simulink model "LQR_crane"  (R2024b)
settings: Solver=ode15s  StartTime=0.0  StopTime=100  MaxStep=1e-3  RelTol=1e-3
values from neighbouring files (symbols this model uses):
  A = [MatriX11, MatriX12, MatriX13, MatriX14, MatriX15, MatriX16,  MatriX17, MatriX18, MatriX19, MatriX110, MatriX111, MatriX112 ... (first row only)    [jacobian_crane.m]    (also in matrices_jacobian.mat = [0 0 0 0 0 0 1 0 0 0 0 0 ... (144 elements, 12x12)]; matrices_jacobian_better.mat = [0 0 0 0 0 0 1 0 0 0 0 0 ... (144 elements, 12x12)])
  B = [0.00067268568898 0 0 0 -0.00401196580412 0 0 0 0 0 0 0 ... (48 elements, 12x4)]    [Bjacobian.mat]    (also in jacobian_crane.m = [B11, B12, B13, B14; matrices_jacobian.mat; matrices_jacobian_better.mat)
  C = eye(12)    [Extended_kalman_filter.m]    (also in crane_control_21_05.m; crane_controlling.m; crane_inner_loop.m = [ 2*d6*dd6*m - dth2*l_B^2*m*sin(2*th2) - dth3*l_J^2*m*sin(2*)
  C_dague = pinv(C)    [crane_control_21_05.m]
  D = zeros(12, 4)    [Extended_kalman_filter.m]    (also in crane_control_21_05.m; crane_controlling.m)
  K = lqr(Ai, Bi, Q, R)    [Extended_kalman_filter.m]    (also in crane_control_21_05.m = lqr(A, B, Q, R); crane_controlling.m = lqr(A, B, Q, R))
  Matrix_pos = diag([zeros(1, floor(12/2)), ones(1, ceil(12/2))])    [crane_control_21_05.m]
  Matrix_speed = [eye(6, 12); zeros(6, 12)]    [crane_control_21_05.m]
  N = K*C_dague - B_dague * A * C_dague    [crane_control_21_05.m]
  x0 = x_eq    [crane_PFL_22_05.m]    (also in crane_control_21_05.m)
  x_d = [0 ... (first row only)    [crane_PFL_22_05.m]    (also in crane_control_21_05.m; crane_controlling.m)
  x_eq = xtraj(1:end, i)    [Extended_kalman_filter.m]    (also in crane_PFL_22_05.m = [zeros(6,1); pi/6; pi/3; -pi/6; 0.5; 0; 0]; crane_control_21_05.m = [zeros(6,1); pi/6; pi/3; -pi/6; 0.5; 0; 0]; crane_controlling.m = [zeros(6,1); pi/6; pi/3; -pi/6; 0.5; 0; 0]; jacobian_crane.m = [zeros(6,1); pi/6; pi/3; -pi/6; 0.5; 0; 0])
settings Model: Creator=david  LastModifiedBy=joelm
settings RTWCC: GPUComputeCapability=3.5

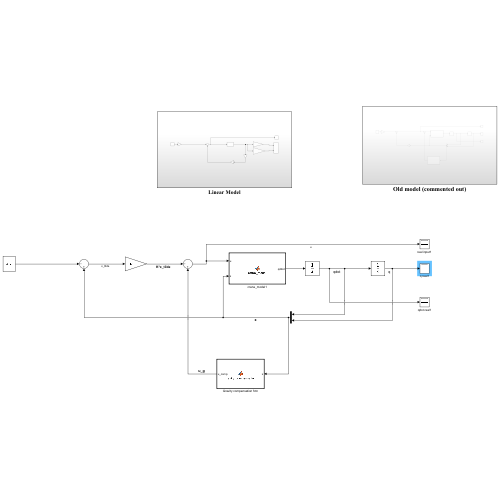
[thumbnail: Simulink's stored preview of the top-level diagram]
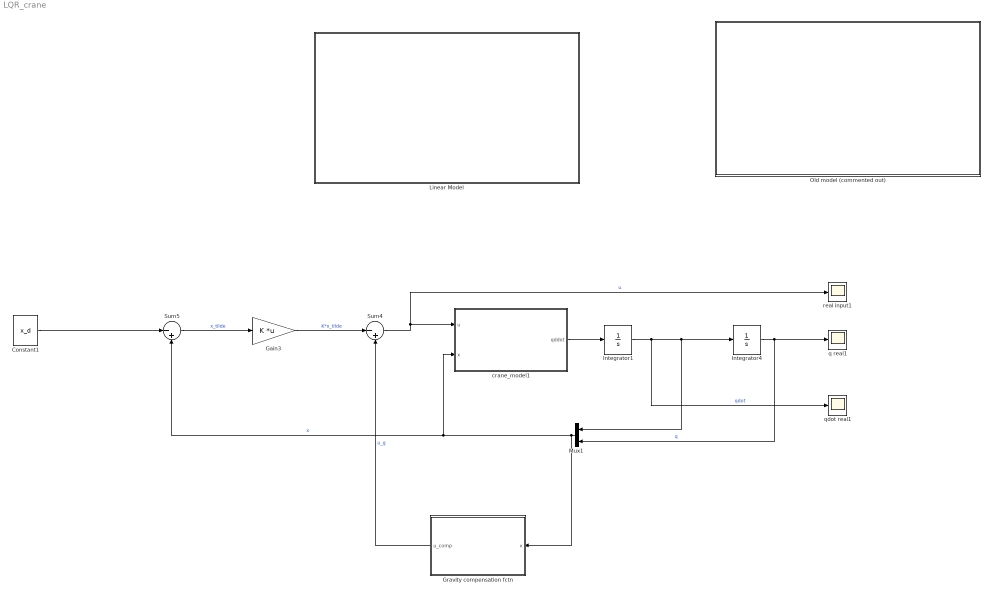
== system LQR_crane ==
  Constant1 : Constant  Value=x_d
  Gain3 : Gain  Gain=K  Multiplication=Matrix(K*u)
  Gravity compensation fctn : MATLAB Function  TreatAsAtomicUnit=on
  Integrator1 : Integrator  InitialCondition=zeros(6,1)
  Integrator4 : Integrator  InitialCondition=x_eq(7:12)
  Linear Model : Subsystem
  Mux1 : Mux  Inputs=2
  Old model (commented out) : Subsystem
  Sum4 : Sum  Inputs=|-+
  Sum5 : Sum  Inputs=|-+
  crane_model1 : MATLAB Function  TreatAsAtomicUnit=on
  q real1 : Scope
  qdot real1 : Scope
  real input1 : Scope
  wires:
  Gravity compensation fctn/1(u_comp) -> Sum4/2  "u_g"
  Sum4/1 -> crane_model1/1(u), real input1/1  "u"
  Integrator4/1 -> Mux1/2, q real1/1  "q"
  Integrator1/1 -> qdot real1/1, Mux1/1, Integrator4/1  "qdot"
  Mux1/1 -> Gravity compensation fctn/1(x), Sum5/2, crane_model1/2(x)  "x"
  Constant1/1 -> Sum5/1
  crane_model1/1(qddot) -> Integrator1/1
  Sum5/1 -> Gain3/1  "x_tilde"
  Gain3/1 -> Sum4/1  "K*x_tilde"

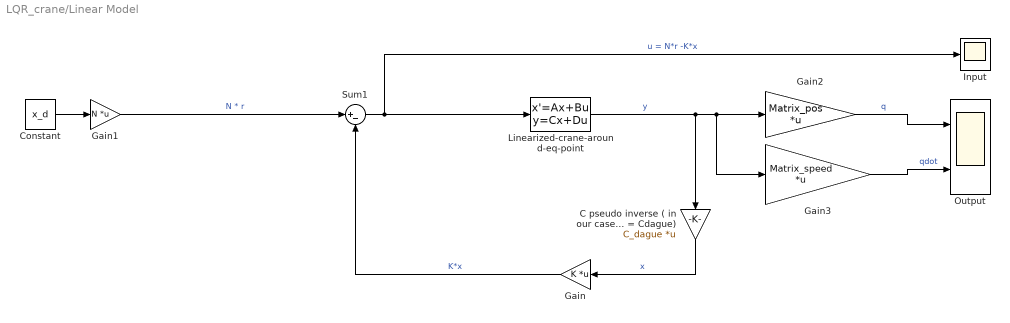
== system LQR_crane/Linear Model ==
  C pseudo inverse ( in our case C is I so = Cdague) : Gain  Gain=C_dague  Multiplication=Matrix(K*u)
  Constant : Constant  Value=x_d
  Gain : Gain  Gain=K  Multiplication=Matrix(K*u)
  Gain1 : Gain  Gain=N  Multiplication=Matrix(K*u)
  Gain2 : Gain  Gain=Matrix_pos  Multiplication=Matrix(K*u)
  Gain3 : Gain  Gain=Matrix_speed  Multiplication=Matrix(K*u)
  Input : Scope
  Linearized-crane-around-eq-point : StateSpace  A=A  B=B  C=C  D=D  InitialCondition=x0
  Output : Scope  NumInputPorts=2
  Sum1 : Sum  Inputs=|+-
  wires:
  Gain/1 -> Sum1/2  "K*x"
  C pseudo inverse ( in our case C is I so = Cdague)/1 -> Gain/1  "x"
  Sum1/1 -> Input/1, Linearized-crane-around-eq-point/1  "u = N*r -K*x"
  Linearized-crane-around-eq-point/1 -> Gain3/1, Gain2/1, C pseudo inverse ( in our case C is I so = Cdague)/1  "y"
  Gain1/1 -> Sum1/1  "N * r"
  Constant/1 -> Gain1/1
  Gain2/1 -> Output/1  "q"
  Gain3/1 -> Output/2  "qdot"

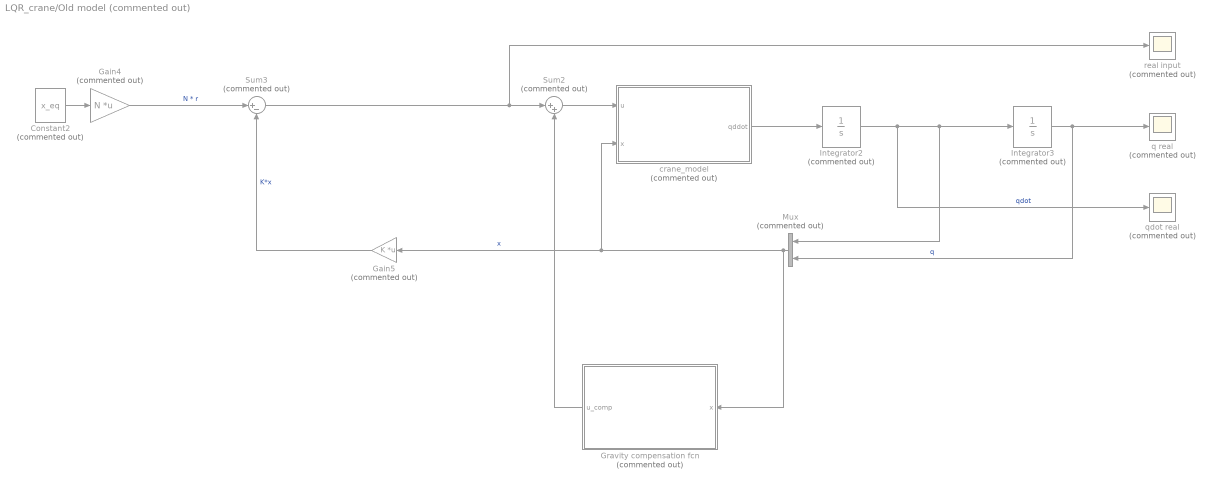
== system LQR_crane/Old model (commented out) ==
  Constant2 : Constant  Commented=on  Value=x_eq
  Gain4 : Gain  Commented=on  Gain=N  Multiplication=Matrix(K*u)
  Gain5 : Gain  Commented=on  Gain=K  Multiplication=Matrix(K*u)
  Gravity compensation fcn : MATLAB Function  Commented=on  TreatAsAtomicUnit=on
  Integrator2 : Integrator  Commented=on  InitialCondition=zeros(6,1)
  Integrator3 : Integrator  Commented=on  InitialCondition=x_eq(7:12)
  Mux : Mux  Commented=on  Inputs=2
  Sum2 : Sum  Commented=on  Inputs=|++
  Sum3 : Sum  Commented=on  Inputs=|+-
  crane_model : MATLAB Function  Commented=on  TreatAsAtomicUnit=on
  q real : Scope  Commented=on
  qdot real : Scope  Commented=on
  real input : Scope  Commented=on
  wires:
  Constant2/1 -> Gain4/1
  Gain5/1 -> Sum3/2  "K*x"
  Sum3/1 -> Sum2/1, real input/1
  Gain4/1 -> Sum3/1  "N * r"
  Mux/1 -> Gravity compensation fcn/1(x), Gain5/1, crane_model/2(x)  "x"
  Integrator3/1 -> Mux/2, q real/1  "q"
  Integrator2/1 -> qdot real/1, Mux/1, Integrator3/1  "qdot"
  Sum2/1 -> crane_model/1(u)
  crane_model/1(qddot) -> Integrator2/1
  Gravity compensation fcn/1(u_comp) -> Sum2/2

== matlab function LQR_crane/Old model (commented out)/Gravity compensation fcn ==
  data: x input; u_comp output
function u_comp = gravity_compensation(x)

I_tot=250;   l_B=2.5;     m_B=300;     I_B=156.25;     l_J=2;     m_J=250;     I_J=85;     g=9.81;       m=90;
  
q = x(7:12);

th1 = q(1);
th2 = q(2);
th3 = q(3);
d6  = q(4);
th4 = q(5);
th5 = q(6);
    
u_comp = [                               0;
(g*l_B*cos(th2)*(2*m + m_B + 2*m_J))/2;
     (g*l_J*cos(th3)*(2*m + m_J))/2;
             -g*m*cos(th4)*cos(th5)];

end

== matlab function LQR_crane/Gravity compensation fctn ==
  data: x input; u_comp output
function u_comp = gravity_compensation(x)

I_tot=250;   l_B=2.5;     m_B=300;     I_B=156.25;     l_J=2;     m_J=250;     I_J=85;     g=9.81;       m=90;
  
q = x(7:12);

th1 = q(1);
th2 = q(2);
th3 = q(3);
d6  = q(4);
th4 = q(5);
th5 = q(6);
    
u_comp = [                               0;
(g*l_B*cos(th2)*(2*m + m_B + 2*m_J))/2;
     (g*l_J*cos(th3)*(2*m + m_J))/2;
             -g*m*cos(th4)*cos(th5)];

end

== matlab function LQR_crane/crane_model1 ==
  data: u input; qddot output; x input
function qddot = crane_model(u, x)



    I_tot=250;   l_B=2.5;     m_B=300;     I_B=156.25;     l_J=2;     m_J=250;     I_J=85;     g=9.81;       m=90;
    
    qdot = x(1:6);
    q = x(7:12); % Function changed for consistency, one state vector with [qdot; q]

    th1 = q(1);
    th2 = q(2);
    th3 = q(3);
    d6  = q(4);
    th4 = q(5);
    th5 = q(6);
    
    
    dth1 = qdot(1);
    dth2 = qdot(2);
    dth3 = qdot(3);
    dd6  =  qdot(4);
    dth4 = qdot(5);
    dth5  =qdot(6);
    
    
    
    M = [ I_tot + d6^2*m + l_B^2*m*cos(th2)^2 + l_J^2*m*cos(th3)^2 + (l_B^2*m_B*cos(th2)^2)/4 + l_B^2*m_J*cos(th2)^2 + (l_J^2*m_J*cos(th3)^2)/4 - d6^2*m*cos(th4)^2*cos(th5)^2 + 2*l_B*l_J*m*cos(th2)*cos(th3) + l_B*l_J*m_J*cos(th2)*cos(th3) + 2*d6*l_B*m*cos(th2)*sin(th5) + 2*d6*l_J*m*cos(th3)*sin(th5),                          d6*l_B*m*cos(th5)*sin(th2)*sin(th4),                          d6*l_J*m*cos(th5)*sin(th3)*sin(th4),            m*cos(th5)*sin(th4)*(l_B*cos(th2) + l_J*cos(th3)), d6*m*cos(th4)*cos(th5)*(l_B*cos(th2) + l_J*cos(th3) + d6*sin(th5)), -d6*m*sin(th4)*(d6 + l_B*cos(th2)*sin(th5) + l_J*cos(th3)*sin(th5));
                                                                                                                                                                                                                                                                     d6*l_B*m*cos(th5)*sin(th2)*sin(th4),                    I_B + l_B^2*m + (l_B^2*m_B)/4 + l_B^2*m_J,                       (l_B*l_J*cos(th2 - th3)*(2*m + m_J))/2, - l_B*m*sin(th2)*sin(th5) - l_B*m*cos(th2)*cos(th4)*cos(th5),                                d6*l_B*m*cos(th2)*cos(th5)*sin(th4),          -d6*l_B*m*(cos(th5)*sin(th2) - cos(th2)*cos(th4)*sin(th5));
                                                                                                                                                                                                                                                                    d6*l_J*m*cos(th5)*sin(th3)*sin(th4),                       (l_B*l_J*cos(th2 - th3)*(2*m + m_J))/2,                                I_J + l_J^2*m + (l_J^2*m_J)/4, - l_J*m*sin(th3)*sin(th5) - l_J*m*cos(th3)*cos(th4)*cos(th5),                                d6*l_J*m*cos(th3)*cos(th5)*sin(th4),          -d6*l_J*m*(cos(th5)*sin(th3) - cos(th3)*cos(th4)*sin(th5));
                                                                                                                                                                                                                                                      m*cos(th5)*sin(th4)*(l_B*cos(th2) + l_J*cos(th3)), - l_B*m*sin(th2)*sin(th5) - l_B*m*cos(th2)*cos(th4)*cos(th5), - l_J*m*sin(th3)*sin(th5) - l_J*m*cos(th3)*cos(th4)*cos(th5),                                                            m,                                                                  0,                                                                   0;
                                                                                                                                                                                                                                     d6*m*cos(th4)*cos(th5)*(l_B*cos(th2) + l_J*cos(th3) + d6*sin(th5)),                          d6*l_B*m*cos(th2)*cos(th5)*sin(th4),                          d6*l_J*m*cos(th3)*cos(th5)*sin(th4),                                                            0,                                           -d6^2*m*(sin(th5)^2 - 1),                                                                   0;
                                                                                                                                                                                                                                    -d6*m*sin(th4)*(d6 + l_B*cos(th2)*sin(th5) + l_J*cos(th3)*sin(th5)),   -d6*l_B*m*(cos(th5)*sin(th2) - cos(th2)*cos(th4)*sin(th5)),   -d6*l_J*m*(cos(th5)*sin(th3) - cos(th3)*cos(th4)*sin(th5)),                                                            0,                                                                  0,                                                              d6^2*m];
                                                                                                                                                                                                                            
    
    % Small regularization
    %%%%%%%%%%%%%%%%%%%%%%%%%%%%%%%%%%%%%%%
    
    C = [ 2*d6*dd6*m - dth2*l_B^2*m*sin(2*th2) - dth3*l_J^2*m*sin(2*th3) - (dth2*l_B^2*m_B*sin(2*th2))/4 - dth2*l_B^2*m_J*sin(2*th2) - (dth3*l_J^2*m_J*sin(2*th3))/4 - 2*d6*dd6*m*cos(th4)^2*cos(th5)^2 + 2*dd6*l_B*m*cos(th2)*sin(th5) + 2*dd6*l_J*m*cos(th3)*sin(th5) + 2*d6*dth5*l_B*m*cos(th2)*cos(th5) + 2*d6*dth5*l_J*m*cos(th3)*cos(th5) - 2*dth2*l_B*l_J*m*cos(th3)*sin(th2) - 2*dth3*l_B*l_J*m*cos(th2)*sin(th3) - dth2*l_B*l_J*m_J*cos(th3)*sin(th2) - dth3*l_B*l_J*m_J*cos(th2)*sin(th3) - 2*d6*dth2*l_B*m*sin(th2)*sin(th5) - 2*d6*dth3*l_J*m*sin(th3)*sin(th5) + 2*d6^2*dth4*m*cos(th4)*cos(th5)^2*sin(th4) + 2*d6^2*dth5*m*cos(th4)^2*cos(th5)*sin(th5),                                                                                                                                                                                                                                                         dd6*l_B*m*cos(th5)*sin(th2)*sin(th4) + d6*dth2*l_B*m*cos(th2)*cos(th5)*sin(th4) + d6*dth4*l_B*m*cos(th4)*cos(th5)*sin(th2) - d6*dth5*l_B*m*sin(th2)*sin(th4)*sin(th5),                                                                                                                                                                                                                                                         dd6*l_J*m*cos(th5)*sin(th3)*sin(th4) + d6*dth3*l_J*m*cos(th3)*cos(th5)*sin(th4) + d6*dth4*l_J*m*cos(th4)*cos(th5)*sin(th3) - d6*dth5*l_J*m*sin(th3)*sin(th4)*sin(th5),       dth4*l_B*m*cos(th2)*cos(th4)*cos(th5) + dth4*l_J*m*cos(th3)*cos(th4)*cos(th5) - dth2*l_B*m*cos(th5)*sin(th2)*sin(th4) - dth5*l_B*m*cos(th2)*sin(th4)*sin(th5) - dth3*l_J*m*cos(th5)*sin(th3)*sin(th4) - dth5*l_J*m*cos(th3)*sin(th4)*sin(th5), 2*d6^2*dth5*m*cos(th4)*cos(th5)^2 - d6^2*dth5*m*cos(th4) + dd6*l_B*m*cos(th2)*cos(th4)*cos(th5) + dd6*l_J*m*cos(th3)*cos(th4)*cos(th5) + 2*d6*dd6*m*cos(th4)*cos(th5)*sin(th5) - d6^2*dth4*m*cos(th5)*sin(th4)*sin(th5) - d6*dth2*l_B*m*cos(th4)*cos(th5)*sin(th2) - d6*dth4*l_B*m*cos(th2)*cos(th5)*sin(th4) - d6*dth5*l_B*m*cos(th2)*cos(th4)*sin(th5) - d6*dth3*l_J*m*cos(th4)*cos(th5)*sin(th3) - d6*dth4*l_J*m*cos(th3)*cos(th5)*sin(th4) - d6*dth5*l_J*m*cos(th3)*cos(th4)*sin(th5), d6*dth2*l_B*m*sin(th2)*sin(th4)*sin(th5) - d6^2*dth4*m*cos(th4) - dd6*l_B*m*cos(th2)*sin(th4)*sin(th5) - dd6*l_J*m*cos(th3)*sin(th4)*sin(th5) - d6*dth4*l_B*m*cos(th2)*cos(th4)*sin(th5) - d6*dth5*l_B*m*cos(th2)*cos(th5)*sin(th4) - d6*dth4*l_J*m*cos(th3)*cos(th4)*sin(th5) - d6*dth5*l_J*m*cos(th3)*cos(th5)*sin(th4) - 2*d6*dd6*m*sin(th4) + d6*dth3*l_J*m*sin(th3)*sin(th4)*sin(th5);
                                                                                                                                                                                                                                                     (dth1*l_B^2*m*sin(2*th2))/2 + (dth1*l_B^2*m_B*sin(2*th2))/8 + (dth1*l_B^2*m_J*sin(2*th2))/2 + (3*dd6*l_B*m*cos(th5)*sin(th2)*sin(th4))/2 + dth1*l_B*l_J*m*cos(th3)*sin(th2) + (dth1*l_B*l_J*m_J*cos(th3)*sin(th2))/2 + d6*dth1*l_B*m*sin(th2)*sin(th5) + (d6*dth2*l_B*m*cos(th2)*cos(th5)*sin(th4))/2 + (3*d6*dth4*l_B*m*cos(th4)*cos(th5)*sin(th2))/2 - (3*d6*dth5*l_B*m*sin(th2)*sin(th4)*sin(th5))/2, (dd6*l_B*m*cos(th2)*sin(th5))/2 - (dd6*l_B*m*cos(th4)*cos(th5)*sin(th2))/2 + (d6*dth5*l_B*m*cos(th2)*cos(th5))/2 - (dth3*l_B*l_J*m*cos(th2)*sin(th3))/2 + (dth3*l_B*l_J*m*cos(th3)*sin(th2))/2 - (dth3*l_B*l_J*m_J*cos(th2)*sin(th3))/4 + (dth3*l_B*l_J*m_J*cos(th3)*sin(th2))/4 - (d6*dth1*l_B*m*cos(th2)*cos(th5)*sin(th4))/2 + (d6*dth4*l_B*m*cos(th5)*sin(th2)*sin(th4))/2 + (d6*dth5*l_B*m*cos(th4)*sin(th2)*sin(th5))/2,                                                                                                                                                                                                                                                                                                                                                                       -(l_B*l_J*sin(th2 - th3)*(dth2 - 2*dth3)*(2*m + m_J))/4,             (dth2*l_B*m*cos(th4)*cos(th5)*sin(th2))/2 - dth5*l_B*m*cos(th5)*sin(th2) - (dth2*l_B*m*cos(th2)*sin(th5))/2 + dth4*l_B*m*cos(th2)*cos(th5)*sin(th4) + dth5*l_B*m*cos(th2)*cos(th4)*sin(th5) + (dth1*l_B*m*cos(th5)*sin(th2)*sin(th4))/2,                                                                                                                                                                                                                                                                  dd6*l_B*m*cos(th2)*cos(th5)*sin(th4) + d6*dth4*l_B*m*cos(th2)*cos(th4)*cos(th5) + (d6*dth1*l_B*m*cos(th4)*cos(th5)*sin(th2))/2 - (d6*dth2*l_B*m*cos(th5)*sin(th2)*sin(th4))/2 - d6*dth5*l_B*m*cos(th2)*sin(th4)*sin(th5),                                                             dd6*l_B*m*cos(th2)*cos(th4)*sin(th5) - dd6*l_B*m*cos(th5)*sin(th2) - (d6*dth2*l_B*m*cos(th2)*cos(th5))/2 + d6*dth5*l_B*m*sin(th2)*sin(th5) + d6*dth5*l_B*m*cos(th2)*cos(th4)*cos(th5) - (d6*dth2*l_B*m*cos(th4)*sin(th2)*sin(th5))/2 - d6*dth4*l_B*m*cos(th2)*sin(th4)*sin(th5) - (d6*dth1*l_B*m*sin(th2)*sin(th4)*sin(th5))/2;
                                                                                                                                                                                                                                                                                     (dth1*l_J^2*m*sin(2*th3))/2 + (dth1*l_J^2*m_J*sin(2*th3))/8 + (3*dd6*l_J*m*cos(th5)*sin(th3)*sin(th4))/2 + dth1*l_B*l_J*m*cos(th2)*sin(th3) + (dth1*l_B*l_J*m_J*cos(th2)*sin(th3))/2 + d6*dth1*l_J*m*sin(th3)*sin(th5) + (d6*dth3*l_J*m*cos(th3)*cos(th5)*sin(th4))/2 + (3*d6*dth4*l_J*m*cos(th4)*cos(th5)*sin(th3))/2 - (3*d6*dth5*l_J*m*sin(th3)*sin(th4)*sin(th5))/2,                                                                                                                                                                                                                                                                                                                                                                       -(l_B*l_J*sin(th2 - th3)*(2*m + m_J)*(2*dth2 - dth3))/4, (dd6*l_J*m*cos(th3)*sin(th5))/2 - (dd6*l_J*m*cos(th4)*cos(th5)*sin(th3))/2 + (d6*dth5*l_J*m*cos(th3)*cos(th5))/2 + (dth2*l_B*l_J*m*cos(th2)*sin(th3))/2 - (dth2*l_B*l_J*m*cos(th3)*sin(th2))/2 + (dth2*l_B*l_J*m_J*cos(th2)*sin(th3))/4 - (dth2*l_B*l_J*m_J*cos(th3)*sin(th2))/4 - (d6*dth1*l_J*m*cos(th3)*cos(th5)*sin(th4))/2 + (d6*dth4*l_J*m*cos(th5)*sin(th3)*sin(th4))/2 + (d6*dth5*l_J*m*cos(th4)*sin(th3)*sin(th5))/2,             (dth3*l_J*m*cos(th4)*cos(th5)*sin(th3))/2 - dth5*l_J*m*cos(th5)*sin(th3) - (dth3*l_J*m*cos(th3)*sin(th5))/2 + dth4*l_J*m*cos(th3)*cos(th5)*sin(th4) + dth5*l_J*m*cos(th3)*cos(th4)*sin(th5) + (dth1*l_J*m*cos(th5)*sin(th3)*sin(th4))/2,                                                                                                                                                                                                                                                                  dd6*l_J*m*cos(th3)*cos(th5)*sin(th4) + d6*dth4*l_J*m*cos(th3)*cos(th4)*cos(th5) + (d6*dth1*l_J*m*cos(th4)*cos(th5)*sin(th3))/2 - (d6*dth3*l_J*m*cos(th5)*sin(th3)*sin(th4))/2 - d6*dth5*l_J*m*cos(th3)*sin(th4)*sin(th5),                                                             dd6*l_J*m*cos(th3)*cos(th4)*sin(th5) - dd6*l_J*m*cos(th5)*sin(th3) - (d6*dth3*l_J*m*cos(th3)*cos(th5))/2 + d6*dth5*l_J*m*sin(th3)*sin(th5) + d6*dth5*l_J*m*cos(th3)*cos(th4)*cos(th5) - (d6*dth3*l_J*m*cos(th4)*sin(th3)*sin(th5))/2 - d6*dth4*l_J*m*cos(th3)*sin(th4)*sin(th5) - (d6*dth1*l_J*m*sin(th3)*sin(th4)*sin(th5))/2;
                                                                                                                                                                                                           d6*dth5*m*sin(th4) - d6*dth1*m + d6*dth1*m*cos(th4)^2*cos(th5)^2 - dth1*l_B*m*cos(th2)*sin(th5) - dth1*l_J*m*cos(th3)*sin(th5) + (dth4*l_B*m*cos(th2)*cos(th4)*cos(th5))/2 + (dth4*l_J*m*cos(th3)*cos(th4)*cos(th5))/2 - d6*dth4*m*cos(th4)*cos(th5)*sin(th5) - (3*dth2*l_B*m*cos(th5)*sin(th2)*sin(th4))/2 - (dth5*l_B*m*cos(th2)*sin(th4)*sin(th5))/2 - (3*dth3*l_J*m*cos(th5)*sin(th3)*sin(th4))/2 - (dth5*l_J*m*cos(th3)*sin(th4)*sin(th5))/2,                                                                                                                                                                                   dth2*l_B*m*cos(th4)*cos(th5)*sin(th2) - (dth5*l_B*m*cos(th5)*sin(th2))/2 - dth2*l_B*m*cos(th2)*sin(th5) + (dth4*l_B*m*cos(th2)*cos(th5)*sin(th4))/2 + (dth5*l_B*m*cos(th2)*cos(th4)*sin(th5))/2 - (dth1*l_B*m*cos(th5)*sin(th2)*sin(th4))/2,                                                                                                                                                                                   dth3*l_J*m*cos(th4)*cos(th5)*sin(th3) - (dth5*l_J*m*cos(th5)*sin(th3))/2 - dth3*l_J*m*cos(th3)*sin(th5) + (dth4*l_J*m*cos(th3)*cos(th5)*sin(th4))/2 + (dth5*l_J*m*cos(th3)*cos(th4)*sin(th5))/2 - (dth1*l_J*m*cos(th5)*sin(th3)*sin(th4))/2,                                                                                                                                                                                                                                                   0,                                                                                                                                                                                                                                                                                                    -(m*cos(th5)*(2*d6*dth4*cos(th5) + dth1*l_B*cos(th2)*cos(th4) + dth1*l_J*cos(th3)*cos(th4) + 2*d6*dth1*cos(th4)*sin(th5) + dth2*l_B*cos(th2)*sin(th4) + dth3*l_J*cos(th3)*sin(th4)))/2,                                                                                                       d6*dth1*m*sin(th4) - d6*dth5*m + (dth2*l_B*m*cos(th5)*sin(th2))/2 + (dth3*l_J*m*cos(th5)*sin(th3))/2 - (dth2*l_B*m*cos(th2)*cos(th4)*sin(th5))/2 - (dth3*l_J*m*cos(th3)*cos(th4)*sin(th5))/2 + (dth1*l_B*m*cos(th2)*sin(th4)*sin(th5))/2 + (dth1*l_J*m*cos(th3)*sin(th4)*sin(th5))/2;
                                                                            2*d6^2*dth5*m*cos(th4)*cos(th5)^2 - (d6^2*dth5*m*cos(th4))/2 + (dd6*l_B*m*cos(th2)*cos(th4)*cos(th5))/2 + (dd6*l_J*m*cos(th3)*cos(th4)*cos(th5))/2 + 2*d6*dd6*m*cos(th4)*cos(th5)*sin(th5) - (d6^2*dth4*m*cos(th5)*sin(th4)*sin(th5))/2 - d6^2*dth1*m*cos(th4)*cos(th5)^2*sin(th4) - (3*d6*dth2*l_B*m*cos(th4)*cos(th5)*sin(th2))/2 - (d6*dth4*l_B*m*cos(th2)*cos(th5)*sin(th4))/2 - (d6*dth5*l_B*m*cos(th2)*cos(th4)*sin(th5))/2 - (3*d6*dth3*l_J*m*cos(th4)*cos(th5)*sin(th3))/2 - (d6*dth4*l_J*m*cos(th3)*cos(th5)*sin(th4))/2 - (d6*dth5*l_J*m*cos(th3)*cos(th4)*sin(th5))/2,                                                                                                                                                                                              (dd6*l_B*m*cos(th2)*cos(th5)*sin(th4))/2 + (d6*dth4*l_B*m*cos(th2)*cos(th4)*cos(th5))/2 - (d6*dth1*l_B*m*cos(th4)*cos(th5)*sin(th2))/2 - d6*dth2*l_B*m*cos(th5)*sin(th2)*sin(th4) - (d6*dth5*l_B*m*cos(th2)*sin(th4)*sin(th5))/2,                                                                                                                                                                                              (dd6*l_J*m*cos(th3)*cos(th5)*sin(th4))/2 + (d6*dth4*l_J*m*cos(th3)*cos(th4)*cos(th5))/2 - (d6*dth1*l_J*m*cos(th4)*cos(th5)*sin(th3))/2 - d6*dth3*l_J*m*cos(th5)*sin(th3)*sin(th4) - (d6*dth5*l_J*m*cos(th3)*sin(th4)*sin(th5))/2,                                                                                                                 -(m*cos(th5)*(dth1*l_B*cos(th2)*cos(th4) + dth1*l_J*cos(th3)*cos(th4) + dth2*l_B*cos(th2)*sin(th4) + dth3*l_J*cos(th3)*sin(th4)))/2,                                                                                                                                                                                                                                                                                   (d6*m*cos(th5)*(4*dd6*cos(th5) - 4*d6*dth5*sin(th5) - dth2*l_B*cos(th2)*cos(th4) - dth3*l_J*cos(th3)*cos(th4) + dth1*l_B*cos(th2)*sin(th4) + dth1*l_J*cos(th3)*sin(th4) + d6*dth1*sin(th4)*sin(th5)))/2,                                                                                                                                                                                                        (d6*m*(d6*dth1*cos(th4) + dth1*l_B*cos(th2)*cos(th4)*sin(th5) + dth1*l_J*cos(th3)*cos(th4)*sin(th5) + dth2*l_B*cos(th2)*sin(th4)*sin(th5) + dth3*l_J*cos(th3)*sin(th4)*sin(th5)))/2;
                                                                         (3*d6*dth2*l_B*m*sin(th2)*sin(th4)*sin(th5))/2 - (d6^2*dth4*m*cos(th4))/2 - d6^2*dth4*m*cos(th4)*cos(th5)^2 - (dd6*l_B*m*cos(th2)*sin(th4)*sin(th5))/2 - (dd6*l_J*m*cos(th3)*sin(th4)*sin(th5))/2 - d6*dth1*l_B*m*cos(th2)*cos(th5) - d6*dth1*l_J*m*cos(th3)*cos(th5) - d6^2*dth1*m*cos(th4)^2*cos(th5)*sin(th5) - (d6*dth4*l_B*m*cos(th2)*cos(th4)*sin(th5))/2 - (d6*dth5*l_B*m*cos(th2)*cos(th5)*sin(th4))/2 - (d6*dth4*l_J*m*cos(th3)*cos(th4)*sin(th5))/2 - (d6*dth5*l_J*m*cos(th3)*cos(th5)*sin(th4))/2 - 2*d6*dd6*m*sin(th4) + (3*d6*dth3*l_J*m*sin(th3)*sin(th4)*sin(th5))/2,                                                                                    (dd6*l_B*m*cos(th2)*cos(th4)*sin(th5))/2 - (dd6*l_B*m*cos(th5)*sin(th2))/2 - d6*dth2*l_B*m*cos(th2)*cos(th5) + (d6*dth5*l_B*m*sin(th2)*sin(th5))/2 + (d6*dth5*l_B*m*cos(th2)*cos(th4)*cos(th5))/2 - d6*dth2*l_B*m*cos(th4)*sin(th2)*sin(th5) - (d6*dth4*l_B*m*cos(th2)*sin(th4)*sin(th5))/2 + (d6*dth1*l_B*m*sin(th2)*sin(th4)*sin(th5))/2,                                                                                    (dd6*l_J*m*cos(th3)*cos(th4)*sin(th5))/2 - (dd6*l_J*m*cos(th5)*sin(th3))/2 - d6*dth3*l_J*m*cos(th3)*cos(th5) + (d6*dth5*l_J*m*sin(th3)*sin(th5))/2 + (d6*dth5*l_J*m*cos(th3)*cos(th4)*cos(th5))/2 - d6*dth3*l_J*m*cos(th4)*sin(th3)*sin(th5) - (d6*dth4*l_J*m*cos(th3)*sin(th4)*sin(th5))/2 + (d6*dth1*l_J*m*sin(th3)*sin(th4)*sin(th5))/2, (dth2*l_B*m*cos(th5)*sin(th2))/2 + (dth3*l_J*m*cos(th5)*sin(th3))/2 - (dth2*l_B*m*cos(th2)*cos(th4)*sin(th5))/2 - (dth3*l_J*m*cos(th3)*cos(th4)*sin(th5))/2 + (dth1*l_B*m*cos(th2)*sin(th4)*sin(th5))/2 + (dth1*l_J*m*cos(th3)*sin(th4)*sin(th5))/2,                                                                                                                                                                                                    (d6^2*dth1*m*cos(th4))/2 - d6^2*dth1*m*cos(th4)*cos(th5)^2 + d6^2*dth4*m*cos(th5)*sin(th5) + (d6*dth1*l_B*m*cos(th2)*cos(th4)*sin(th5))/2 + (d6*dth1*l_J*m*cos(th3)*cos(th4)*sin(th5))/2 + (d6*dth2*l_B*m*cos(th2)*sin(th4)*sin(th5))/2 + (d6*dth3*l_J*m*cos(th3)*sin(th4)*sin(th5))/2,                                                                                                                                                        -(d6*m*(dth2*l_B*sin(th2)*sin(th5) - 4*dd6 + dth3*l_J*sin(th3)*sin(th5) + dth2*l_B*cos(th2)*cos(th4)*cos(th5) + dth3*l_J*cos(th3)*cos(th4)*cos(th5) - dth1*l_B*cos(th2)*cos(th5)*sin(th4) - dth1*l_J*cos(th3)*cos(th5)*sin(th4)))/2];
    
    
    %%%%%%%%%%%%%%%%%%%%%%%%%%%%%%%%%%%%%%%%%%%%%
    
    G = [                                0;
    (g*l_B*cos(th2)*(2*m + m_B + 2*m_J))/2;
         (g*l_J*cos(th3)*(2*m + m_J))/2;
                 -g*m*cos(th4)*cos(th5);
               d6*g*m*cos(th5)*sin(th4);
               d6*g*m*cos(th4)*sin(th5)];

    U = [u(1); u(2); u(3); u(4); 0; 0];     %%%the last two dof are the angles of the swaying cable and are not actuable

    
    % Compute right-hand side
    rhs = -C*qdot - G + U;
    
    % Solve for qddot 
    qddot = M \ rhs;
    
    

end

== matlab function LQR_crane/Old model (commented out)/crane_model ==
  data: u input; qddot output; x input
function qddot = crane_model(u, x)



    I_tot=250;   l_B=2.5;     m_B=300;     I_B=156.25;     l_J=2;     m_J=250;     I_J=85;     g=9.81;       m=90;
    
    qdot = x(1:6);
    q = x(7:12); % Function changed for consistency, one state vector with [qdot; q]

    th1 = q(1);
    th2 = q(2);
    th3 = q(3);
    d6  = q(4);
    th4 = q(5);
    th5 = q(6);
    
    
    dth1 = qdot(1);
    dth2 = qdot(2);
    dth3 = qdot(3);
    dd6  =  qdot(4);
    dth4 = qdot(5);
    dth5  =qdot(6);
    
    
    
    M = [ I_tot + d6^2*m + l_B^2*m*cos(th2)^2 + l_J^2*m*cos(th3)^2 + (l_B^2*m_B*cos(th2)^2)/4 + l_B^2*m_J*cos(th2)^2 + (l_J^2*m_J*cos(th3)^2)/4 - d6^2*m*cos(th4)^2*cos(th5)^2 + 2*l_B*l_J*m*cos(th2)*cos(th3) + l_B*l_J*m_J*cos(th2)*cos(th3) + 2*d6*l_B*m*cos(th2)*sin(th5) + 2*d6*l_J*m*cos(th3)*sin(th5),                          d6*l_B*m*cos(th5)*sin(th2)*sin(th4),                          d6*l_J*m*cos(th5)*sin(th3)*sin(th4),            m*cos(th5)*sin(th4)*(l_B*cos(th2) + l_J*cos(th3)), d6*m*cos(th4)*cos(th5)*(l_B*cos(th2) + l_J*cos(th3) + d6*sin(th5)), -d6*m*sin(th4)*(d6 + l_B*cos(th2)*sin(th5) + l_J*cos(th3)*sin(th5));
                                                                                                                                                                                                                                                                     d6*l_B*m*cos(th5)*sin(th2)*sin(th4),                    I_B + l_B^2*m + (l_B^2*m_B)/4 + l_B^2*m_J,                       (l_B*l_J*cos(th2 - th3)*(2*m + m_J))/2, - l_B*m*sin(th2)*sin(th5) - l_B*m*cos(th2)*cos(th4)*cos(th5),                                d6*l_B*m*cos(th2)*cos(th5)*sin(th4),          -d6*l_B*m*(cos(th5)*sin(th2) - cos(th2)*cos(th4)*sin(th5));
                                                                                                                                                                                                                                                                    d6*l_J*m*cos(th5)*sin(th3)*sin(th4),                       (l_B*l_J*cos(th2 - th3)*(2*m + m_J))/2,                                I_J + l_J^2*m + (l_J^2*m_J)/4, - l_J*m*sin(th3)*sin(th5) - l_J*m*cos(th3)*cos(th4)*cos(th5),                                d6*l_J*m*cos(th3)*cos(th5)*sin(th4),          -d6*l_J*m*(cos(th5)*sin(th3) - cos(th3)*cos(th4)*sin(th5));
                                                                                                                                                                                                                                                      m*cos(th5)*sin(th4)*(l_B*cos(th2) + l_J*cos(th3)), - l_B*m*sin(th2)*sin(th5) - l_B*m*cos(th2)*cos(th4)*cos(th5), - l_J*m*sin(th3)*sin(th5) - l_J*m*cos(th3)*cos(th4)*cos(th5),                                                            m,                                                                  0,                                                                   0;
                                                                                                                                                                                                                                     d6*m*cos(th4)*cos(th5)*(l_B*cos(th2) + l_J*cos(th3) + d6*sin(th5)),                          d6*l_B*m*cos(th2)*cos(th5)*sin(th4),                          d6*l_J*m*cos(th3)*cos(th5)*sin(th4),                                                            0,                                           -d6^2*m*(sin(th5)^2 - 1),                                                                   0;
                                                                                                                                                                                                                                    -d6*m*sin(th4)*(d6 + l_B*cos(th2)*sin(th5) + l_J*cos(th3)*sin(th5)),   -d6*l_B*m*(cos(th5)*sin(th2) - cos(th2)*cos(th4)*sin(th5)),   -d6*l_J*m*(cos(th5)*sin(th3) - cos(th3)*cos(th4)*sin(th5)),                                                            0,                                                                  0,                                                              d6^2*m];
                                                                                                                                                                                                                            
    
    % Small regularization
    %%%%%%%%%%%%%%%%%%%%%%%%%%%%%%%%%%%%%%%
    
    C = [ 2*d6*dd6*m - dth2*l_B^2*m*sin(2*th2) - dth3*l_J^2*m*sin(2*th3) - (dth2*l_B^2*m_B*sin(2*th2))/4 - dth2*l_B^2*m_J*sin(2*th2) - (dth3*l_J^2*m_J*sin(2*th3))/4 - 2*d6*dd6*m*cos(th4)^2*cos(th5)^2 + 2*dd6*l_B*m*cos(th2)*sin(th5) + 2*dd6*l_J*m*cos(th3)*sin(th5) + 2*d6*dth5*l_B*m*cos(th2)*cos(th5) + 2*d6*dth5*l_J*m*cos(th3)*cos(th5) - 2*dth2*l_B*l_J*m*cos(th3)*sin(th2) - 2*dth3*l_B*l_J*m*cos(th2)*sin(th3) - dth2*l_B*l_J*m_J*cos(th3)*sin(th2) - dth3*l_B*l_J*m_J*cos(th2)*sin(th3) - 2*d6*dth2*l_B*m*sin(th2)*sin(th5) - 2*d6*dth3*l_J*m*sin(th3)*sin(th5) + 2*d6^2*dth4*m*cos(th4)*cos(th5)^2*sin(th4) + 2*d6^2*dth5*m*cos(th4)^2*cos(th5)*sin(th5),                                                                                                                                                                                                                                                         dd6*l_B*m*cos(th5)*sin(th2)*sin(th4) + d6*dth2*l_B*m*cos(th2)*cos(th5)*sin(th4) + d6*dth4*l_B*m*cos(th4)*cos(th5)*sin(th2) - d6*dth5*l_B*m*sin(th2)*sin(th4)*sin(th5),                                                                                                                                                                                                                                                         dd6*l_J*m*cos(th5)*sin(th3)*sin(th4) + d6*dth3*l_J*m*cos(th3)*cos(th5)*sin(th4) + d6*dth4*l_J*m*cos(th4)*cos(th5)*sin(th3) - d6*dth5*l_J*m*sin(th3)*sin(th4)*sin(th5),       dth4*l_B*m*cos(th2)*cos(th4)*cos(th5) + dth4*l_J*m*cos(th3)*cos(th4)*cos(th5) - dth2*l_B*m*cos(th5)*sin(th2)*sin(th4) - dth5*l_B*m*cos(th2)*sin(th4)*sin(th5) - dth3*l_J*m*cos(th5)*sin(th3)*sin(th4) - dth5*l_J*m*cos(th3)*sin(th4)*sin(th5), 2*d6^2*dth5*m*cos(th4)*cos(th5)^2 - d6^2*dth5*m*cos(th4) + dd6*l_B*m*cos(th2)*cos(th4)*cos(th5) + dd6*l_J*m*cos(th3)*cos(th4)*cos(th5) + 2*d6*dd6*m*cos(th4)*cos(th5)*sin(th5) - d6^2*dth4*m*cos(th5)*sin(th4)*sin(th5) - d6*dth2*l_B*m*cos(th4)*cos(th5)*sin(th2) - d6*dth4*l_B*m*cos(th2)*cos(th5)*sin(th4) - d6*dth5*l_B*m*cos(th2)*cos(th4)*sin(th5) - d6*dth3*l_J*m*cos(th4)*cos(th5)*sin(th3) - d6*dth4*l_J*m*cos(th3)*cos(th5)*sin(th4) - d6*dth5*l_J*m*cos(th3)*cos(th4)*sin(th5), d6*dth2*l_B*m*sin(th2)*sin(th4)*sin(th5) - d6^2*dth4*m*cos(th4) - dd6*l_B*m*cos(th2)*sin(th4)*sin(th5) - dd6*l_J*m*cos(th3)*sin(th4)*sin(th5) - d6*dth4*l_B*m*cos(th2)*cos(th4)*sin(th5) - d6*dth5*l_B*m*cos(th2)*cos(th5)*sin(th4) - d6*dth4*l_J*m*cos(th3)*cos(th4)*sin(th5) - d6*dth5*l_J*m*cos(th3)*cos(th5)*sin(th4) - 2*d6*dd6*m*sin(th4) + d6*dth3*l_J*m*sin(th3)*sin(th4)*sin(th5);
                                                                                                                                                                                                                                                     (dth1*l_B^2*m*sin(2*th2))/2 + (dth1*l_B^2*m_B*sin(2*th2))/8 + (dth1*l_B^2*m_J*sin(2*th2))/2 + (3*dd6*l_B*m*cos(th5)*sin(th2)*sin(th4))/2 + dth1*l_B*l_J*m*cos(th3)*sin(th2) + (dth1*l_B*l_J*m_J*cos(th3)*sin(th2))/2 + d6*dth1*l_B*m*sin(th2)*sin(th5) + (d6*dth2*l_B*m*cos(th2)*cos(th5)*sin(th4))/2 + (3*d6*dth4*l_B*m*cos(th4)*cos(th5)*sin(th2))/2 - (3*d6*dth5*l_B*m*sin(th2)*sin(th4)*sin(th5))/2, (dd6*l_B*m*cos(th2)*sin(th5))/2 - (dd6*l_B*m*cos(th4)*cos(th5)*sin(th2))/2 + (d6*dth5*l_B*m*cos(th2)*cos(th5))/2 - (dth3*l_B*l_J*m*cos(th2)*sin(th3))/2 + (dth3*l_B*l_J*m*cos(th3)*sin(th2))/2 - (dth3*l_B*l_J*m_J*cos(th2)*sin(th3))/4 + (dth3*l_B*l_J*m_J*cos(th3)*sin(th2))/4 - (d6*dth1*l_B*m*cos(th2)*cos(th5)*sin(th4))/2 + (d6*dth4*l_B*m*cos(th5)*sin(th2)*sin(th4))/2 + (d6*dth5*l_B*m*cos(th4)*sin(th2)*sin(th5))/2,                                                                                                                                                                                                                                                                                                                                                                       -(l_B*l_J*sin(th2 - th3)*(dth2 - 2*dth3)*(2*m + m_J))/4,             (dth2*l_B*m*cos(th4)*cos(th5)*sin(th2))/2 - dth5*l_B*m*cos(th5)*sin(th2) - (dth2*l_B*m*cos(th2)*sin(th5))/2 + dth4*l_B*m*cos(th2)*cos(th5)*sin(th4) + dth5*l_B*m*cos(th2)*cos(th4)*sin(th5) + (dth1*l_B*m*cos(th5)*sin(th2)*sin(th4))/2,                                                                                                                                                                                                                                                                  dd6*l_B*m*cos(th2)*cos(th5)*sin(th4) + d6*dth4*l_B*m*cos(th2)*cos(th4)*cos(th5) + (d6*dth1*l_B*m*cos(th4)*cos(th5)*sin(th2))/2 - (d6*dth2*l_B*m*cos(th5)*sin(th2)*sin(th4))/2 - d6*dth5*l_B*m*cos(th2)*sin(th4)*sin(th5),                                                             dd6*l_B*m*cos(th2)*cos(th4)*sin(th5) - dd6*l_B*m*cos(th5)*sin(th2) - (d6*dth2*l_B*m*cos(th2)*cos(th5))/2 + d6*dth5*l_B*m*sin(th2)*sin(th5) + d6*dth5*l_B*m*cos(th2)*cos(th4)*cos(th5) - (d6*dth2*l_B*m*cos(th4)*sin(th2)*sin(th5))/2 - d6*dth4*l_B*m*cos(th2)*sin(th4)*sin(th5) - (d6*dth1*l_B*m*sin(th2)*sin(th4)*sin(th5))/2;
                                                                                                                                                                                                                                                                                     (dth1*l_J^2*m*sin(2*th3))/2 + (dth1*l_J^2*m_J*sin(2*th3))/8 + (3*dd6*l_J*m*cos(th5)*sin(th3)*sin(th4))/2 + dth1*l_B*l_J*m*cos(th2)*sin(th3) + (dth1*l_B*l_J*m_J*cos(th2)*sin(th3))/2 + d6*dth1*l_J*m*sin(th3)*sin(th5) + (d6*dth3*l_J*m*cos(th3)*cos(th5)*sin(th4))/2 + (3*d6*dth4*l_J*m*cos(th4)*cos(th5)*sin(th3))/2 - (3*d6*dth5*l_J*m*sin(th3)*sin(th4)*sin(th5))/2,                                                                                                                                                                                                                                                                                                                                                                       -(l_B*l_J*sin(th2 - th3)*(2*m + m_J)*(2*dth2 - dth3))/4, (dd6*l_J*m*cos(th3)*sin(th5))/2 - (dd6*l_J*m*cos(th4)*cos(th5)*sin(th3))/2 + (d6*dth5*l_J*m*cos(th3)*cos(th5))/2 + (dth2*l_B*l_J*m*cos(th2)*sin(th3))/2 - (dth2*l_B*l_J*m*cos(th3)*sin(th2))/2 + (dth2*l_B*l_J*m_J*cos(th2)*sin(th3))/4 - (dth2*l_B*l_J*m_J*cos(th3)*sin(th2))/4 - (d6*dth1*l_J*m*cos(th3)*cos(th5)*sin(th4))/2 + (d6*dth4*l_J*m*cos(th5)*sin(th3)*sin(th4))/2 + (d6*dth5*l_J*m*cos(th4)*sin(th3)*sin(th5))/2,             (dth3*l_J*m*cos(th4)*cos(th5)*sin(th3))/2 - dth5*l_J*m*cos(th5)*sin(th3) - (dth3*l_J*m*cos(th3)*sin(th5))/2 + dth4*l_J*m*cos(th3)*cos(th5)*sin(th4) + dth5*l_J*m*cos(th3)*cos(th4)*sin(th5) + (dth1*l_J*m*cos(th5)*sin(th3)*sin(th4))/2,                                                                                                                                                                                                                                                                  dd6*l_J*m*cos(th3)*cos(th5)*sin(th4) + d6*dth4*l_J*m*cos(th3)*cos(th4)*cos(th5) + (d6*dth1*l_J*m*cos(th4)*cos(th5)*sin(th3))/2 - (d6*dth3*l_J*m*cos(th5)*sin(th3)*sin(th4))/2 - d6*dth5*l_J*m*cos(th3)*sin(th4)*sin(th5),                                                             dd6*l_J*m*cos(th3)*cos(th4)*sin(th5) - dd6*l_J*m*cos(th5)*sin(th3) - (d6*dth3*l_J*m*cos(th3)*cos(th5))/2 + d6*dth5*l_J*m*sin(th3)*sin(th5) + d6*dth5*l_J*m*cos(th3)*cos(th4)*cos(th5) - (d6*dth3*l_J*m*cos(th4)*sin(th3)*sin(th5))/2 - d6*dth4*l_J*m*cos(th3)*sin(th4)*sin(th5) - (d6*dth1*l_J*m*sin(th3)*sin(th4)*sin(th5))/2;
                                                                                                                                                                                                           d6*dth5*m*sin(th4) - d6*dth1*m + d6*dth1*m*cos(th4)^2*cos(th5)^2 - dth1*l_B*m*cos(th2)*sin(th5) - dth1*l_J*m*cos(th3)*sin(th5) + (dth4*l_B*m*cos(th2)*cos(th4)*cos(th5))/2 + (dth4*l_J*m*cos(th3)*cos(th4)*cos(th5))/2 - d6*dth4*m*cos(th4)*cos(th5)*sin(th5) - (3*dth2*l_B*m*cos(th5)*sin(th2)*sin(th4))/2 - (dth5*l_B*m*cos(th2)*sin(th4)*sin(th5))/2 - (3*dth3*l_J*m*cos(th5)*sin(th3)*sin(th4))/2 - (dth5*l_J*m*cos(th3)*sin(th4)*sin(th5))/2,                                                                                                                                                                                   dth2*l_B*m*cos(th4)*cos(th5)*sin(th2) - (dth5*l_B*m*cos(th5)*sin(th2))/2 - dth2*l_B*m*cos(th2)*sin(th5) + (dth4*l_B*m*cos(th2)*cos(th5)*sin(th4))/2 + (dth5*l_B*m*cos(th2)*cos(th4)*sin(th5))/2 - (dth1*l_B*m*cos(th5)*sin(th2)*sin(th4))/2,                                                                                                                                                                                   dth3*l_J*m*cos(th4)*cos(th5)*sin(th3) - (dth5*l_J*m*cos(th5)*sin(th3))/2 - dth3*l_J*m*cos(th3)*sin(th5) + (dth4*l_J*m*cos(th3)*cos(th5)*sin(th4))/2 + (dth5*l_J*m*cos(th3)*cos(th4)*sin(th5))/2 - (dth1*l_J*m*cos(th5)*sin(th3)*sin(th4))/2,                                                                                                                                                                                                                                                   0,                                                                                                                                                                                                                                                                                                    -(m*cos(th5)*(2*d6*dth4*cos(th5) + dth1*l_B*cos(th2)*cos(th4) + dth1*l_J*cos(th3)*cos(th4) + 2*d6*dth1*cos(th4)*sin(th5) + dth2*l_B*cos(th2)*sin(th4) + dth3*l_J*cos(th3)*sin(th4)))/2,                                                                                                       d6*dth1*m*sin(th4) - d6*dth5*m + (dth2*l_B*m*cos(th5)*sin(th2))/2 + (dth3*l_J*m*cos(th5)*sin(th3))/2 - (dth2*l_B*m*cos(th2)*cos(th4)*sin(th5))/2 - (dth3*l_J*m*cos(th3)*cos(th4)*sin(th5))/2 + (dth1*l_B*m*cos(th2)*sin(th4)*sin(th5))/2 + (dth1*l_J*m*cos(th3)*sin(th4)*sin(th5))/2;
                                                                            2*d6^2*dth5*m*cos(th4)*cos(th5)^2 - (d6^2*dth5*m*cos(th4))/2 + (dd6*l_B*m*cos(th2)*cos(th4)*cos(th5))/2 + (dd6*l_J*m*cos(th3)*cos(th4)*cos(th5))/2 + 2*d6*dd6*m*cos(th4)*cos(th5)*sin(th5) - (d6^2*dth4*m*cos(th5)*sin(th4)*sin(th5))/2 - d6^2*dth1*m*cos(th4)*cos(th5)^2*sin(th4) - (3*d6*dth2*l_B*m*cos(th4)*cos(th5)*sin(th2))/2 - (d6*dth4*l_B*m*cos(th2)*cos(th5)*sin(th4))/2 - (d6*dth5*l_B*m*cos(th2)*cos(th4)*sin(th5))/2 - (3*d6*dth3*l_J*m*cos(th4)*cos(th5)*sin(th3))/2 - (d6*dth4*l_J*m*cos(th3)*cos(th5)*sin(th4))/2 - (d6*dth5*l_J*m*cos(th3)*cos(th4)*sin(th5))/2,                                                                                                                                                                                              (dd6*l_B*m*cos(th2)*cos(th5)*sin(th4))/2 + (d6*dth4*l_B*m*cos(th2)*cos(th4)*cos(th5))/2 - (d6*dth1*l_B*m*cos(th4)*cos(th5)*sin(th2))/2 - d6*dth2*l_B*m*cos(th5)*sin(th2)*sin(th4) - (d6*dth5*l_B*m*cos(th2)*sin(th4)*sin(th5))/2,                                                                                                                                                                                              (dd6*l_J*m*cos(th3)*cos(th5)*sin(th4))/2 + (d6*dth4*l_J*m*cos(th3)*cos(th4)*cos(th5))/2 - (d6*dth1*l_J*m*cos(th4)*cos(th5)*sin(th3))/2 - d6*dth3*l_J*m*cos(th5)*sin(th3)*sin(th4) - (d6*dth5*l_J*m*cos(th3)*sin(th4)*sin(th5))/2,                                                                                                                 -(m*cos(th5)*(dth1*l_B*cos(th2)*cos(th4) + dth1*l_J*cos(th3)*cos(th4) + dth2*l_B*cos(th2)*sin(th4) + dth3*l_J*cos(th3)*sin(th4)))/2,                                                                                                                                                                                                                                                                                   (d6*m*cos(th5)*(4*dd6*cos(th5) - 4*d6*dth5*sin(th5) - dth2*l_B*cos(th2)*cos(th4) - dth3*l_J*cos(th3)*cos(th4) + dth1*l_B*cos(th2)*sin(th4) + dth1*l_J*cos(th3)*sin(th4) + d6*dth1*sin(th4)*sin(th5)))/2,                                                                                                                                                                                                        (d6*m*(d6*dth1*cos(th4) + dth1*l_B*cos(th2)*cos(th4)*sin(th5) + dth1*l_J*cos(th3)*cos(th4)*sin(th5) + dth2*l_B*cos(th2)*sin(th4)*sin(th5) + dth3*l_J*cos(th3)*sin(th4)*sin(th5)))/2;
                                                                         (3*d6*dth2*l_B*m*sin(th2)*sin(th4)*sin(th5))/2 - (d6^2*dth4*m*cos(th4))/2 - d6^2*dth4*m*cos(th4)*cos(th5)^2 - (dd6*l_B*m*cos(th2)*sin(th4)*sin(th5))/2 - (dd6*l_J*m*cos(th3)*sin(th4)*sin(th5))/2 - d6*dth1*l_B*m*cos(th2)*cos(th5) - d6*dth1*l_J*m*cos(th3)*cos(th5) - d6^2*dth1*m*cos(th4)^2*cos(th5)*sin(th5) - (d6*dth4*l_B*m*cos(th2)*cos(th4)*sin(th5))/2 - (d6*dth5*l_B*m*cos(th2)*cos(th5)*sin(th4))/2 - (d6*dth4*l_J*m*cos(th3)*cos(th4)*sin(th5))/2 - (d6*dth5*l_J*m*cos(th3)*cos(th5)*sin(th4))/2 - 2*d6*dd6*m*sin(th4) + (3*d6*dth3*l_J*m*sin(th3)*sin(th4)*sin(th5))/2,                                                                                    (dd6*l_B*m*cos(th2)*cos(th4)*sin(th5))/2 - (dd6*l_B*m*cos(th5)*sin(th2))/2 - d6*dth2*l_B*m*cos(th2)*cos(th5) + (d6*dth5*l_B*m*sin(th2)*sin(th5))/2 + (d6*dth5*l_B*m*cos(th2)*cos(th4)*cos(th5))/2 - d6*dth2*l_B*m*cos(th4)*sin(th2)*sin(th5) - (d6*dth4*l_B*m*cos(th2)*sin(th4)*sin(th5))/2 + (d6*dth1*l_B*m*sin(th2)*sin(th4)*sin(th5))/2,                                                                                    (dd6*l_J*m*cos(th3)*cos(th4)*sin(th5))/2 - (dd6*l_J*m*cos(th5)*sin(th3))/2 - d6*dth3*l_J*m*cos(th3)*cos(th5) + (d6*dth5*l_J*m*sin(th3)*sin(th5))/2 + (d6*dth5*l_J*m*cos(th3)*cos(th4)*cos(th5))/2 - d6*dth3*l_J*m*cos(th4)*sin(th3)*sin(th5) - (d6*dth4*l_J*m*cos(th3)*sin(th4)*sin(th5))/2 + (d6*dth1*l_J*m*sin(th3)*sin(th4)*sin(th5))/2, (dth2*l_B*m*cos(th5)*sin(th2))/2 + (dth3*l_J*m*cos(th5)*sin(th3))/2 - (dth2*l_B*m*cos(th2)*cos(th4)*sin(th5))/2 - (dth3*l_J*m*cos(th3)*cos(th4)*sin(th5))/2 + (dth1*l_B*m*cos(th2)*sin(th4)*sin(th5))/2 + (dth1*l_J*m*cos(th3)*sin(th4)*sin(th5))/2,                                                                                                                                                                                                    (d6^2*dth1*m*cos(th4))/2 - d6^2*dth1*m*cos(th4)*cos(th5)^2 + d6^2*dth4*m*cos(th5)*sin(th5) + (d6*dth1*l_B*m*cos(th2)*cos(th4)*sin(th5))/2 + (d6*dth1*l_J*m*cos(th3)*cos(th4)*sin(th5))/2 + (d6*dth2*l_B*m*cos(th2)*sin(th4)*sin(th5))/2 + (d6*dth3*l_J*m*cos(th3)*sin(th4)*sin(th5))/2,                                                                                                                                                        -(d6*m*(dth2*l_B*sin(th2)*sin(th5) - 4*dd6 + dth3*l_J*sin(th3)*sin(th5) + dth2*l_B*cos(th2)*cos(th4)*cos(th5) + dth3*l_J*cos(th3)*cos(th4)*cos(th5) - dth1*l_B*cos(th2)*cos(th5)*sin(th4) - dth1*l_J*cos(th3)*cos(th5)*sin(th4)))/2];
    
    
    %%%%%%%%%%%%%%%%%%%%%%%%%%%%%%%%%%%%%%%%%%%%%
    
    G = [                                0;
    (g*l_B*cos(th2)*(2*m + m_B + 2*m_J))/2;
         (g*l_J*cos(th3)*(2*m + m_J))/2;
                 -g*m*cos(th4)*cos(th5);
               d6*g*m*cos(th5)*sin(th4);
               d6*g*m*cos(th4)*sin(th5)];

    U = [u(1); u(2); u(3); u(4); 0; 0];     %%%the last two dof are the angles of the swaying cable and are not actuable

    
    % Compute right-hand side
    rhs = -C*qdot - G + U;
    
    % Solve for qddot 
    qddot = M \ rhs;
    
    

end
